simulink model "STEVE_Simulations"  (R2024b)
settings: Solver=VariableStepAuto  StartTime=0.0  StopTime=10.0  RelTol=1e-3
libraries: aerolibanim x1
settings Model: Creator=jonno  LastModifiedBy=jonno

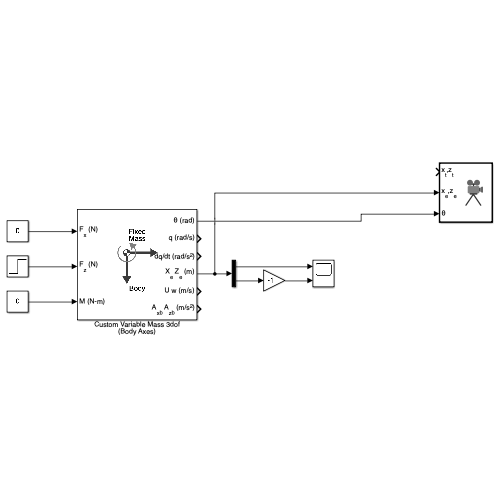
[thumbnail: Simulink's stored preview of the top-level diagram]
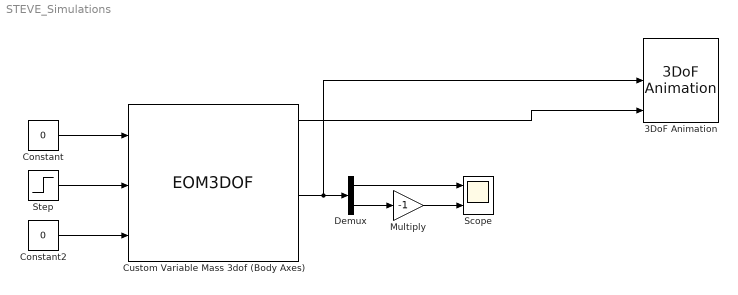
== system STEVE_Simulations ==
  3DoF Animation : aerolibanim/3DoF Animation  u1=[0 5000 -2000 2000 -5050 -3050]  u2=0.05  u3=1.0  u5=Fly alongside  u6=[2000 500 -3150]  u7=10  u8=on
  Constant : Constant  Value=0
  Constant2 : Constant  Value=0
  Custom Variable Mass 3dof (Body Axes) : EOM3DOF  v_ini=0
  Demux : Demux  Outputs=2
  Multiply : Gain  Gain=-1
  Scope : Scope  NumInputPorts=2
  Step : Step  Before=-50  After=0  SampleTime=0
  wires:
  Constant/1 -> Custom Variable Mass 3dof (Body Axes)/1
  Step/1 -> Custom Variable Mass 3dof (Body Axes)/2
  Constant2/1 -> Custom Variable Mass 3dof (Body Axes)/3
  Custom Variable Mass 3dof (Body Axes)/4 -> 3DoF Animation/2, Demux/1
  Demux/1 -> Scope/1
  Demux/2 -> Multiply/1
  Multiply/1 -> Scope/2
  Custom Variable Mass 3dof (Body Axes)/1 -> 3DoF Animation/3
